simulink library "Engine_Lib_org"  (Simulink 10.0)
settings: Solver=ode45  StartTime=0.0  StopTime=10.0  RelTol=1e-3  EnableMultiTasking=on
undefined symbols (not defined in the file): AFR_Table, beta, center, coeffs, DCT_Param, ECP_Table, exponent, ICP_Table, invDG, Load_Table, numterms, polyTerms, S_Table, WendlandNumTerms, width
libraries: fl_lib x8, nesl_utility x6, $bdroot x1, sdl_lib x1
(part 2 of 2)

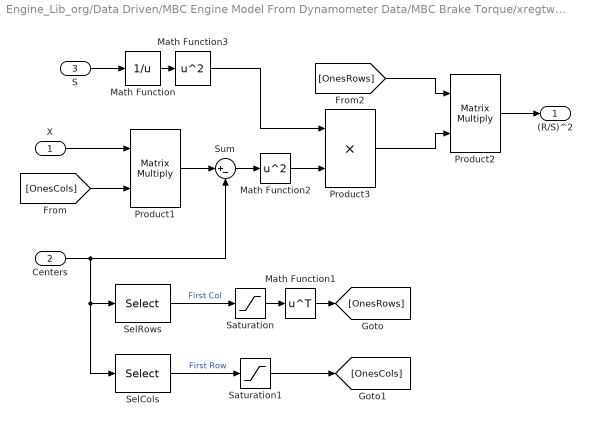
== system Engine_Lib_org/Data Driven/MBC Engine Model From Dynamometer Data/MBC Brake Torque/xregtwostage/RF2/hybridRBFEval/rbfmultiquadricEval/R ==
  X : Inport
  "Centers " : Inport  Port=2
  S : Inport  Port=3
  Math Function : Math  Operator=reciprocal  SaturateOnIntegerOverflow=on
  Math Function1 : Math  Operator=transpose  SaturateOnIntegerOverflow=on
  Math Function2 : Math  Operator=square  SaturateOnIntegerOverflow=on
  Math Function3 : Math  Operator=square  SaturateOnIntegerOverflow=on
  Product1 : Product  Multiplication=Matrix(*)  SaturateOnIntegerOverflow=on  InputSameDT=on  OutDataTypeStr=Inherit: Same as first input
  Product2 : Product  Multiplication=Matrix(*)  SaturateOnIntegerOverflow=on  InputSameDT=on  OutDataTypeStr=Inherit: Same as first input
  Product3 : Product  SaturateOnIntegerOverflow=on  InputSameDT=on  OutDataTypeStr=Inherit: Same as first input
  Saturation : Saturate  UpperLimit=1  LowerLimit=1
  Saturation1 : Saturate  UpperLimit=1  LowerLimit=1
  SelCols : Selector  NumberOfDimensions=2  InputPortWidth=3  IndexOptions=Index vector (dialog),Select all  Indices=1,-1  OutputSizes=1
  SelRows : Selector  NumberOfDimensions=2  InputPortWidth=3  IndexOptions=Select all,Index vector (dialog)  Indices=-1,1  OutputSizes=1
  Sum : Sum  Inputs=|+-  SaturateOnIntegerOverflow=on  InputSameDT=on  OutDataTypeStr=Inherit: Same as first input
  (R/S)^2 : Outport
  wires:
  Math Function2/1 -> Product3/2
  Sum/1 -> Math Function2/1
  Product1/1 -> Sum/1
  X/1 -> Product1/1
  [OnesCols] -> Product1/2
  Math Function1/1 -> [OnesRows]
  SelRows/1 -> Saturation/1  "First Col"
  "Centers "/1 -> Sum/2, SelRows/1, SelCols/1
  S/1 -> Math Function/1
  Math Function/1 -> Math Function3/1
  Saturation/1 -> Math Function1/1
  SelCols/1 -> Saturation1/1  "First Row"
  Saturation1/1 -> [OnesCols]
  Math Function3/1 -> Product3/1
  Product3/1 -> Product2/2
  Product2/1 -> (R/S)^2/1
  [OnesRows] -> Product2/1

== system Engine_Lib_org/Data Driven/MBC Engine Model From Dynamometer Data/MBC Brake Torque/xregtwostage/RF3/hybridRBFEval/rbfmultiquadricEval/MqGlobalWidth ==
  note: If Sigma has more than one width per dimension
      | then y = sqrt ((R/S)^2 +1)
      | otherwise y = S * sqrt ((R/S)^2 +1)
      |
      | This subsystem deals with the global width case.
      | See Multiquadric for thewidth/dim, width/center
      | and width/center/dim cases.
  (R/S)^2 : Inport
  S : Inport  Port=2
  Constant1 : Constant
  Math Function2 : Math  Operator=sqrt  SaturateOnIntegerOverflow=on
  Product : Product  SaturateOnIntegerOverflow=on  InputSameDT=on  OutDataTypeStr=Inherit: Same as first input
  Selector : Selector  NumberOfDimensions=2  IndexOptions=Index vector (dialog),Index vector (dialog)  Indices=1,1  OutputSizes=1
  Sum : Sum  Inputs=++|  SaturateOnIntegerOverflow=on  InputSameDT=on  OutDataTypeStr=Inherit: Same as first input
  P : Outport
  wires:
  Selector/1 -> Product/2
  Product/1 -> P/1
  Math Function2/1 -> Product/1
  Constant1/1 -> Sum/1
  (R/S)^2/1 -> Sum/2
  Sum/1 -> Math Function2/1
  S/1 -> Selector/1

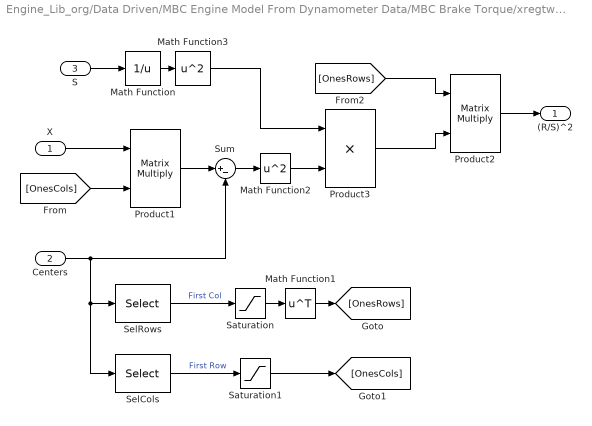
== system Engine_Lib_org/Data Driven/MBC Engine Model From Dynamometer Data/MBC Brake Torque/xregtwostage/RF3/hybridRBFEval/rbfmultiquadricEval/R ==
  X : Inport
  "Centers " : Inport  Port=2
  S : Inport  Port=3
  Math Function : Math  Operator=reciprocal  SaturateOnIntegerOverflow=on
  Math Function1 : Math  Operator=transpose  SaturateOnIntegerOverflow=on
  Math Function2 : Math  Operator=square  SaturateOnIntegerOverflow=on
  Math Function3 : Math  Operator=square  SaturateOnIntegerOverflow=on
  Product1 : Product  Multiplication=Matrix(*)  SaturateOnIntegerOverflow=on  InputSameDT=on  OutDataTypeStr=Inherit: Same as first input
  Product2 : Product  Multiplication=Matrix(*)  SaturateOnIntegerOverflow=on  InputSameDT=on  OutDataTypeStr=Inherit: Same as first input
  Product3 : Product  SaturateOnIntegerOverflow=on  InputSameDT=on  OutDataTypeStr=Inherit: Same as first input
  Saturation : Saturate  UpperLimit=1  LowerLimit=1
  Saturation1 : Saturate  UpperLimit=1  LowerLimit=1
  SelCols : Selector  NumberOfDimensions=2  InputPortWidth=3  IndexOptions=Index vector (dialog),Select all  Indices=1,-1  OutputSizes=1
  SelRows : Selector  NumberOfDimensions=2  InputPortWidth=3  IndexOptions=Select all,Index vector (dialog)  Indices=-1,1  OutputSizes=1
  Sum : Sum  Inputs=|+-  SaturateOnIntegerOverflow=on  InputSameDT=on  OutDataTypeStr=Inherit: Same as first input
  (R/S)^2 : Outport
  wires:
  Math Function2/1 -> Product3/2
  Sum/1 -> Math Function2/1
  Product1/1 -> Sum/1
  X/1 -> Product1/1
  [OnesCols] -> Product1/2
  Math Function1/1 -> [OnesRows]
  SelRows/1 -> Saturation/1  "First Col"
  "Centers "/1 -> Sum/2, SelRows/1, SelCols/1
  S/1 -> Math Function/1
  Math Function/1 -> Math Function3/1
  Saturation/1 -> Math Function1/1
  SelCols/1 -> Saturation1/1  "First Row"
  Saturation1/1 -> [OnesCols]
  Math Function3/1 -> Product3/1
  Product3/1 -> Product2/2
  Product2/1 -> (R/S)^2/1
  [OnesRows] -> Product2/1
